simulink model "lab01"  (R2021a)
settings: Solver=VariableStepAuto  StartTime=0.0  StopTime=10.0  RelTol=1e-3
settings Model: Creator=fantavit  LastModifiedBy=fantavit

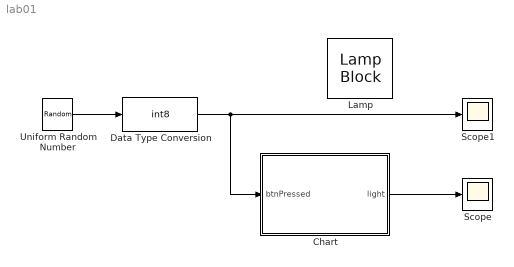
== system lab01 ==
  Chart : Stateflow chart  TreatAsAtomicUnit=on
  Data Type Conversion : DataTypeConversion  OutMin=[0]  OutMax=[1]  OutDataTypeStr=int8
  Lamp : LampBlock
  Scope : Scope
  Scope1 : Scope
  Uniform Random Number : UniformRandomNumber  Minimum=0  Maximum=2  SampleTime=0.1
  wires:
  Chart/1(light) -> Scope/1
  Uniform Random Number/1 -> Data Type Conversion/1
  Data Type Conversion/1 -> Scope1/1, Chart/1(btnPressed)

== stateflow chart lab01/Chart ==
  state ON_BRIGHTER
    entry:
    light = 2;
  state ON
    entry:
    light = 1;
  state OFF
    entry:
    light = 0;
  state BROKEN
    entry:
    light = 0;
  ON_BRIGHTER -> OFF : [btnPressed == 1]
  (default) -> OFF
  ON -> OFF [order 2] : [btnPressed == 1]
  OFF -> ON : [btnPressed == 1]
  ON -> ON_BRIGHTER [order 3] : [duration(btnPressed == 1) < 0.2
      | ]
  ON -> BROKEN [order 1] : [elapsed(sec) >= 1
      | ]
  data: btnPressed input; light output
